simulink model "five_level"  (R2014a)
settings: Solver=ode45  StartTime=0.0  StopTime=0.1  RelTol=1e-3
values from neighbouring files (symbols this model uses):
  f4 = b    [fiv_level.m]
  r4 = c    [fiv_level.m]
  v4 = a    [fiv_level.m]
libraries: powerlib x14
settings Model: Creator=SAMBIT  LastModifiedBy=SAMBIT

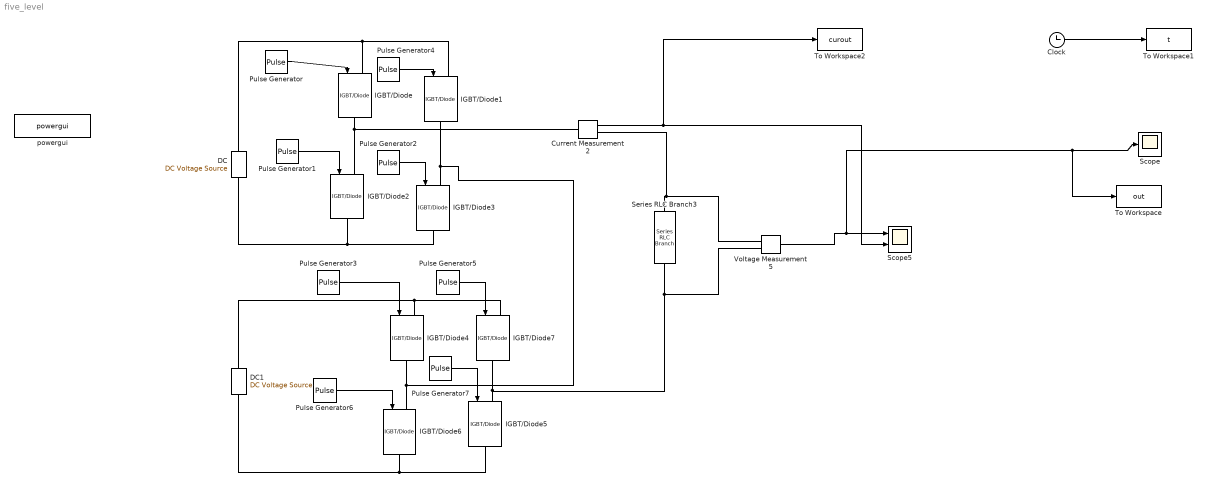
== system five_level ==
  Clock : Clock
  Current Measurement2 : powerlib/Measurements/Current Measurement  PhasorSimulation=off  OutputType=Complex  PSBequivalent=0
  DC : powerlib/Electrical Sources/DC Voltage Source  Amplitude=v4  Measurements=None
  DC1 : powerlib/Electrical Sources/DC Voltage Source  Amplitude=v4  Measurements=None
  IGBT/Diode{,1..7} (8 alike) : powerlib/Power Electronics/IGBT//Diode  Ron=1e-3  Rs=1e5  Cs=inf  Measurements=off
  Pulse Generator : DiscretePulseGenerator  PulseType=Time based  Period=1/f4  PulseWidth=30  PhaseDelay=0.002
  Pulse Generator1 : DiscretePulseGenerator  PulseType=Time based  Period=1/f4  PulseWidth=30  PhaseDelay=0.012
  Pulse Generator2 : DiscretePulseGenerator  PulseType=Time based  Period=1/f4  PulseWidth=30  PhaseDelay=0.002
  Pulse Generator3 : DiscretePulseGenerator  PulseType=Time based  Period=1/f4  PulseWidth=10  PhaseDelay=0.004
  Pulse Generator4 : DiscretePulseGenerator  PulseType=Time based  Period=1/f4  PulseWidth=10  PhaseDelay=0.014
  Pulse Generator5 : DiscretePulseGenerator  PulseType=Time based  Period=1/f4  PulseWidth=30  PhaseDelay=0.012
  Pulse Generator6 : DiscretePulseGenerator  PulseType=Time based  Period=1/f4  PulseWidth=30  PhaseDelay=0.012
  Pulse Generator7 : DiscretePulseGenerator  PulseType=Time based  Period=1/f4  PulseWidth=30  PhaseDelay=0.002
  Scope : Scope
  Scope5 : Scope  NumInputPorts=2
      settings: TimeRange=0.04  YMin=-1~-200  YMax=1~200  SaveName=SPBR_HL_FD  MaxDataPoints=5000000  SampleInput=on  SampleTime=5e-6
  Series RLC Branch3 : powerlib/Elements/Series RLC Branch  LConnTagsString=__new0  RConnTagsString=__new0  BranchType=RL  Resistance=r4  Inductance=0  SetiL0=off  InitialCurrent=0  Capacitance=1e-6  Setx0=off  InitialVoltage=0  Measurements=None
  To Workspace : ToWorkspace  VariableName=out  SampleTime=-1
  To Workspace1 : ToWorkspace  VariableName=t  SampleTime=-1
  To Workspace2 : ToWorkspace  VariableName=curout  SampleTime=-1
  Voltage Measurement5 : powerlib/Measurements/Voltage Measurement  PhasorSimulation=off  OutputType=Complex  PSBequivalent=0
  powergui : powerlib/powergui  Priority=1  SimulationMode=Continuous  SolverType=Tustin  SampleTime=5e-6  frequency=60  SPID=off  DisableSnubberDevices=off  DisableRonSwitches=off  DisableVfSwitches=off  SwTol=0  Interpol=off  DisplayEquations=off  Ts=0  methode=off  frequencyindice=0  Pbase=100e6  ErrMax=1e-4  Iterations=50  UnitsV=kV  UnitsW=MW  FunctionMessages=off  echomessages=off  HookPort=off  EnableUseOfTLC=off  x0status=blocks  RestoreLinks=warning  ResistiveCurrentMeasurement=off  Frange=[0:2:500]  Ylog=off  Xlog=on  ShowGrid=off  save=off  variable=ZData  structure=SPBR_R  ZoomFFT=off  StartTime=0.0  cycles=1  DisplayStyle=1  fundamental=100  FreqAxis=off  MaxFrequency=1000  frequencyindicesteady=1  RmsSteady=1  display=off
  wires:
  Pulse Generator/1 -> IGBT/Diode/1
  Pulse Generator4/1 -> IGBT/Diode1/1
  Pulse Generator1/1 -> IGBT/Diode2/1
  Pulse Generator2/1 -> IGBT/Diode3/1
  Pulse Generator6/1 -> IGBT/Diode6/1
  Pulse Generator3/1 -> IGBT/Diode4/1
  Pulse Generator5/1 -> IGBT/Diode7/1
  Pulse Generator7/1 -> IGBT/Diode5/1
  Current Measurement2/1 -> To Workspace2/1, Scope5/2
  Clock/1 -> To Workspace1/1
  Voltage Measurement5/1 -> To Workspace/1, Scope/1, Scope5/1
  connections:
  DC/LConn1 -- IGBT/Diode3/RConn1 -- IGBT/Diode2/RConn1
  DC/RConn1 -- IGBT/Diode1/LConn1 -- IGBT/Diode/LConn1
  Series RLC Branch3/RConn1 -- Voltage Measurement5/LConn2 -- IGBT/Diode7/RConn1 -- IGBT/Diode5/LConn1
  DC1/LConn1 -- IGBT/Diode6/RConn1 -- IGBT/Diode5/RConn1
  IGBT/Diode1/RConn1 -- IGBT/Diode3/LConn1 -- IGBT/Diode4/RConn1 -- IGBT/Diode6/LConn1
  DC1/RConn1 -- IGBT/Diode7/LConn1 -- IGBT/Diode4/LConn1
  Voltage Measurement5/LConn1 -- Current Measurement2/RConn1 -- Series RLC Branch3/LConn1
  IGBT/Diode/RConn1 -- Current Measurement2/LConn1 -- IGBT/Diode2/LConn1
